simulink model "EcuAppM_StateMachine"  (R2022b)
settings: Solver=FixedStepDiscrete  StartTime=0  StopTime=50  FixedStep=1  RelTol=1e-3  EnableMultiTasking=on
values from neighbouring files (symbols this model uses):
  ECUAPPM_MAX_WAKEUP_SOURCES = mpt.Parameter    [EcuAppM_StateMachine_Param.m]    (also in EcuAppM_StateMachine_Param_For_Safety_Context.m)
  ECUAPPM_VALUE_ZERO = mpt.Parameter    [EcuAppM_StateMachine_Param.m]    (also in EcuAppM_StateMachine_Param_For_Safety_Context.m)
  EcuAppM_WakeupSourcesData = mpt.Parameter    [EcuAppM_StateMachine_Param.m]    (also in EcuAppM_StateMachine_Param_For_Safety_Context.m)
libraries: simulink x3
(part 2 of 2)

== stateflow chart EcuAppM_StateMachine/Subsystem/EcuAppM_StateChart ==
  state EcuAppM_WakeupValidationState
    entry:
    EcuAppM_WakeupValidationTimer = ECUAPPM_VALUE_ZERO;
    EcuAppMInfo.State  = eEcuAppM_WakeupValidation;
    EcuAppMInfo.CurrentJobStatus = ECUAPPM_JOB_IN_PROGRESS;
    EcuAppM_OnWakeupValidationWrapper(EcuAppM_BufferedWakeupSource);
    during:
    EcuAppMInfo.CurrentJobStatus = EcuAppM_ProcessJobStatusWrapper(EcuAppMInfo.State);
    EcuAppM_WakeupValidationTimer = EcuAppM_WakeupValidationTimer + ECUAPPM_PERIOD_MSEC;
    exit:
    EcuAppM_WakeupValidationTimer = ECUAPPM_VALUE_ZERO;
    EcuAppMInfo.CurrentJobStatus = ECUAPPM_JOB_IDLE;
  state EcuAppM_StartOfSleepTransientWrapper [function]
  state EcuAppM_PreGroupActivationState
    entry:
    EcuAppMInfo.State  = eEcuAppM_PreGroupActivation;
    EcuAppMInfo.CurrentJobStatus = ECUAPPM_JOB_IN_PROGRESS;
    EcuAppM_BufferedWakeupSource = EcuAppM_WakeupSource;
    EcuAppM_BufferedWakeupData = EcuAppM_ReadWakeupSourcesConfigData...
    (EcuAppM_BufferedWakeupSource);
    EcuAppM_OnStartupWrapper(EcuAppM_BufferedWakeupSource);
    during:
    EcuAppM_ProcessPreGroupsActivation(PRE_GROUP0);
    EcuAppMInfo.CurrentJobStatus = EcuAppM_ProcessJobStatusWrapper(EcuAppMInfo.State);
    exit:
    EcuAppMInfo.CurrentJobStatus = ECUAPPM_JOB_IDLE;
  state EcuAppM_StartPowerUpSequenceState
    entry:
    EcuAppMInfo.State  = eEcuAppM_StartPowerUpSequence;
    EcuAppMInfo.CurrentJobStatus = ECUAPPM_JOB_IN_PROGRESS;
    EcuAppM_OnPowerSeqStartWrapper(EcuAppMInfo.State);
    during:
    EcuAppMInfo.CurrentJobStatus = EcuAppM_ProcessJobStatusWrapper(EcuAppMInfo.State);
    exit:
    EcuAppMInfo.CurrentJobStatus = ECUAPPM_JOB_IDLE;
  state EcuAppM_ClearWakeupReasonWrapper [function]
  state EcuAppM_StartOfGroupsDeactivationWrapper [function]
  state EcuAppM_OnStartupWrapper(EcuAppM_BufferedWakeupSource) [function]
  state EcuAppM_ReadDataState
    entry:
    EcuAppMInfo.State  = eEcuAppM_ReadDataState;
    exit:
    EcuAppM_BufferedWakeupSource = EcuAppM_WakeupSource;
    state NVMReadallState [parallel]
      entry:
      EcuAppMInfo.CurrentJobStatus = ECUAPPM_JOB_IN_PROGRESS;
      EcuAppM_OnNVMReadAllWrapper(EcuAppM_BufferedWakeupSource);
      during:
      EcuAppMInfo.CurrentJobStatus = EcuAppM_ProcessJobStatusWrapper(EcuAppMInfo.State);
      exit:
      EcuAppMInfo.CurrentJobStatus = ECUAPPM_JOB_IDLE;
      settings: executionOrder=1
    state EcuAppM_PreGroup [parallel]
      entry:
      EcuAppM_ProcessPreGroupsActivation(PRE_GROUP1);
      during:
      EcuAppM_ProcessPreGroupsActivation(PRE_GROUP1);
      settings: executionOrder=2
  state EcuAppM_OnNVMReadAllWrapper(EcuAppM_BufferedWakeupSource) [function]
  state EcuAppM_OnWakeupValidationWrapper(EcuAppM_BufferedWakeupSource) [function]
  state EcuAppM_BackupDataWrapper [function]
  state EcuAppM_GroupsMgmtState
    note: Groups Activation and Deactivation stages summary:
        | 1.Once Deactivation started wake up request is accepted immedietly after ongoing group deactivation.
        | 2.Sleep request is accepted immedietly after ongoing group activation.
        | 3.While Partial wakeup groups are deactivating, if early wakeup comes should not consider immedietly.instead need to allow full deactivation of normal groups. Consider the early wakeup only from EcuAppM_BackupDataState .
        | This is to avoid unnecessary activation of not subcribed groups for that particular wakeup.
    state EcuAppM_GroupsActivationState
      entry:
      EcuAppMInfo.State  = eEcuAppM_GroupsActivation;
      EcuAppMInfo.CurrentJobStatus = ECUAPPM_JOB_IN_PROGRESS;
      during:
      EcuAppM_ProcessGroupsActivation(ECUAPPM_GROUP2,ECUAPPM_MAX_GROUPS - ECUAPPM_VALUE_ONE);
      EcuAppMInfo.CurrentJobStatus = EcuAppM_ProcessJobStatusWrapper(EcuAppMInfo.State);
      exit:
      EcuAppMInfo.CurrentJobStatus = ECUAPPM_JOB_IDLE;
    state EcuAppM_GroupsDeactivationState
      entry:
      EcuAppMInfo.State  = eEcuAppM_GroupsDeactivation;
      EcuAppMInfo.EarlyWakeupCheck = ECUAPPM_FALSE;
      EcuAppMInfo.CurrentJobStatus = ECUAPPM_JOB_IN_PROGRESS;
      EcuAppM_ClearWakeupReasonWrapper();
      EcuAppM_StartOfGroupsDeactivationWrapper();
      during:
      EcuAppM_ProcessGroupsDeactivation(ECUAPPM_MAX_GROUPS - ECUAPPM_VALUE_ONE,ECUAPPM_GROUP2,1);
      EcuAppMInfo.CurrentJobStatus = EcuAppM_ProcessJobStatusWrapper(EcuAppMInfo.State);
      exit:
      EcuAppMInfo.EarlyWakeupCheck = ECUAPPM_FALSE;
      EcuAppMInfo.CurrentJobStatus = ECUAPPM_JOB_IDLE;
    state EcuAppM_EarlyWakeupValidationState
      entry:
      EcuAppM_WakeupValidationTimer = ECUAPPM_VALUE_ZERO;
      EcuAppMInfo.State  = eEcuAppM_WakeupValidation;
      EcuAppMInfo.CurrentJobStatus = ECUAPPM_JOB_IN_PROGRESS;
      EcuAppM_BufferedWakeupData = EcuAppM_ReadWakeupSourcesConfigData(EcuAppM_BufferedWakeupSource);
      EcuAppM_OnWakeupValidationWrapper(EcuAppM_BufferedWakeupSource);
      EcuAppM_ClearWakeupReasonWrapper();
      during:
      EcuAppMInfo.CurrentJobStatus = EcuAppM_ProcessJobStatusWrapper(EcuAppMInfo.State);
      EcuAppM_WakeupValidationTimer = EcuAppM_WakeupValidationTimer + ECUAPPM_PERIOD_MSEC;
      exit:
      EcuAppM_WakeupValidationTimer = ECUAPPM_VALUE_ZERO;
      EcuAppMInfo.CurrentJobStatus = ECUAPPM_JOB_IDLE;
      EcuAppMInfo.EarlyWakeupCheck = ECUAPPM_FALSE;
    (default) -> EcuAppM_GroupsActivationState
    EcuAppM_GroupsActivationState -> EcuAppM_GroupsDeactivationState : [(EcuAppMInfo.CurrentJobStatus == ECUAPPM_JOB_DONE)&&(EcuAppM_CheckActivationStatetimerExpiry() == TRUE)&&...
        |  (EcuAppM_IsGroupsActivationDeactivationAllowed() == ECUAPPM_TRUE)&&(ApplicationSleepState == ECUAPPM_READY_TO_SLEEP)]
    EcuAppM_GroupsDeactivationState -> EcuAppM_EarlyWakeupValidationState [order 1] : [EcuAppMInfo.EarlyWakeupCheck  == ECUAPPM_TRUE]
    EcuAppM_EarlyWakeupValidationState -> EcuAppM_GroupsDeactivationState [order 1] : [(EcuAppMInfo.CurrentJobStatus == ECUAPPM_JOB_FAILED)||...
        |  (EcuAppM_WakeupValidationTimer >= EcuAppM_BufferedWakeupData.validationTime)]
    EcuAppM_EarlyWakeupValidationState -> EcuAppM_GroupsActivationState [order 2] : [(EcuAppMInfo.CurrentJobStatus == ECUAPPM_JOB_DONE)||...
        |  (EcuAppM_BufferedWakeupData.validationTime == ECUAPPM_VALIDATION_TIME_ZERO)]
  state EcuAppM_OnPowerSeqStartWrapper(State) [function]
  state EcuAppM_BufferedDataOutput = EcuAppM_ReadWakeupSourcesConfigData... [function]
    (EcuAppM_BufferedWakeupSource)
  state status = EcuAppM_ProcessJobStatusWrapper(state) [function]
    state status = EcuAppM_ProcessJobStatusFunc(state) [function]
    note: EcuAppM_ProcessJobStatusWrapper Summary:
        |
        | 1. EcuAppM_ProcessJobStatusWrapper Graphical function is used to trigger the EcuAppM_ProcessJobStatusFunc simulink Function.
        | 2.If we are calling EcuAppM_ProcessJobStatusFunc simulink Function With arguments directly, we are facing the error while generating the code(it seems to be a matlab issue).
        | 3.To avoid this, indirectly we are calling the sumulink function with arguments by using Graphical EcuAppM_ProcessJobStatusWrapper function.
        | 4.Calling Simulink function with arguments inside the graphical function is not giving any error hence currently following this approach.
    (default) -> (junction 2651)
    (junction 2651) -> (junction 2652) : {status = EcuAppM_ProcessJobStatusFunc(state)}
  state EcuAppM_BackupDataState
    entry:
    EcuAppMInfo.State  = eEcuAppM_BackupData;
    EcuAppMInfo.CurrentJobStatus = ECUAPPM_JOB_IN_PROGRESS;
    EcuAppM_BackupDataWrapper();
    during:
    EcuAppMInfo.CurrentJobStatus = EcuAppM_ProcessJobStatusWrapper(EcuAppMInfo.State);
    exit:
    EcuAppMInfo.CurrentJobStatus = ECUAPPM_JOB_IDLE;
  state EcuAppM_ProcessPreGroupsActivation(activationstage) [function]
    note: EcuAppM_ProcessPreGroupsActivation Summary:
        |
        | 1. This function will call EcuAppM_GroupsLifeCycleMgr for pre groups activation.Only for wakeup subscribed groups alone.
    (default) -> (junction 3283) : {
        |  pregrp0Index = ECUAPPM_VALUE_ZERO;
        |  pregrp1Index = ECUAPPM_VALUE_ZERO;
        | }
    (junction 3283) -> (junction 3401) [order 1] : [(activationstage == PRE_GROUP0)&&...
        |  (pregrp0Index < ECUAPPM_PREGROUP0_MAX_ELEMENTS)]
    (junction 3401) -> (junction 3284) [order 1] : [EcuAppM_PreGroup0Elements[pregrp0Index] < ECUAPPM_MAX_GROUPS]
    (junction 3284) -> (junction 3285) [order 1] : [((EcuAppM_GroupConfigData[EcuAppM_PreGroup0Elements[pregrp0Index]].wakeupSourceMask & EcuAppM_BufferedWakeupSource) == EcuAppM_BufferedWakeupSource)]
    (junction 3405) -> (junction 3283) : {
        |  pregrp0Index = pregrp0Index + ECUAPPM_VALUE_ONE;
        | }
    (junction 3283) -> (junction 3350) [order 2]
    (junction 3401) -> (junction 3405) [order 2]
    (junction 3284) -> (junction 3286) [order 2]
    (junction 3285) -> (junction 3287) : {
        |   EcuAppM_GroupsLifeCycleMgr(EcuAppM_PreGroup0Elements[pregrp0Index]);
        | }
    (junction 3286) -> (junction 3405)
    (junction 3287) -> (junction 3286)
    (junction 3350) -> (junction 3412) [order 1] : [(activationstage == PRE_GROUP1)&&...
        |  (pregrp1Index < ECUAPPM_PREGROUP1_MAX_ELEMENTS)]
    (junction 3412) -> (junction 3351) [order 1] : [EcuAppM_PreGroup1Elements[pregrp1Index] < ECUAPPM_MAX_GROUPS]
    (junction 3351) -> (junction 3352) [order 1] : [((EcuAppM_GroupConfigData[EcuAppM_PreGroup1Elements[pregrp1Index]].wakeupSourceMask & EcuAppM_BufferedWakeupSource) == EcuAppM_BufferedWakeupSource)]
    (junction 3414) -> (junction 3350) : {
        |  pregrp1Index = pregrp1Index + ECUAPPM_VALUE_ONE;
        | }
    (junction 3350) -> (junction 3362) [order 2]
    (junction 3412) -> (junction 3414) [order 2]
    (junction 3351) -> (junction 3361) [order 2]
    (junction 3352) -> (junction 3360) : {
        |   EcuAppM_GroupsLifeCycleMgr(EcuAppM_PreGroup1Elements[pregrp1Index]);
        | }
    (junction 3361) -> (junction 3414)
    (junction 3360) -> (junction 3361)
  state activationstatus = EcuAppM_IsPreGroupsActivated(activationstage) [function]
    note: EcuAppM_IsPreGroupsActivated Summary:
        |
        | 1. This function is to confirm pre-stages groups are completly activated or not(only particular wakeup subscribed groups status should be checked).
    (default) -> (junction 3223) : {
        |  pregrp0Index = ECUAPPM_VALUE_ZERO;
        |  pregrp1Index = ECUAPPM_VALUE_ZERO;
        | }
    (junction 3336) -> (junction 3419) [order 1] : [EcuAppM_PreGroup0Elements[pregrp0Index] < ECUAPPM_MAX_GROUPS]
    (junction 3419) -> (junction 3224) [order 1] : [((EcuAppM_GroupConfigData[EcuAppM_PreGroup0Elements[pregrp0Index]].wakeupSourceMask & EcuAppM_BufferedWakeupSource) == EcuAppM_BufferedWakeupSource)]
    (junction 3224) -> (junction 3225) [order 1] : [EcuAppM_GroupsInfo.GroupState[EcuAppM_PreGroup0Elements[pregrp0Index]] == eGroup_StateActive]
    (junction 3223) -> (junction 3336) [order 1] : [(activationstage == PRE_GROUP0)&&...
        |  (pregrp0Index < ECUAPPM_PREGROUP0_MAX_ELEMENTS)]
    (junction 3338) -> (junction 3223)
    (junction 3223) -> (junction 3368) [order 2]
    (junction 3336) -> (junction 3338) [order 2] : {
        |  pregrp0Index = pregrp0Index + ECUAPPM_VALUE_ONE;
        |  activationstatus = ECUAPPM_TRUE;
        | }
    (junction 3419) -> (junction 3421) [order 2] : {
        |  pregrp0Index = pregrp0Index + ECUAPPM_VALUE_ONE;
        |  activationstatus = ECUAPPM_TRUE;
        | }
    (junction 3225) -> (junction 3228) : {
        |  pregrp0Index = pregrp0Index + ECUAPPM_VALUE_ONE;
        |  activationstatus = ECUAPPM_TRUE;
        | }
    (junction 3224) -> (junction 3227) [order 2] : {
        |   pregrp0Index = ECUAPPM_PREGROUP0_MAX_ELEMENTS;
        |   activationstatus = ECUAPPM_FALSE;
        | }
    (junction 3421) -> (junction 3338)
    (junction 3227) -> (junction 3421)
    (junction 3228) -> (junction 3227)
    (junction 3368) -> (junction 3424) [order 1] : [(activationstage == PRE_GROUP1)&&...
        |  (pregrp1Index < ECUAPPM_PREGROUP1_MAX_ELEMENTS)]
    (junction 3424) -> (junction 3382) [order 1] : [EcuAppM_PreGroup1Elements[pregrp0Index] < ECUAPPM_MAX_GROUPS]
    (junction 3382) -> (junction 3369) [order 1] : [((EcuAppM_GroupConfigData[EcuAppM_PreGroup1Elements[pregrp0Index]].wakeupSourceMask & EcuAppM_BufferedWakeupSource) == EcuAppM_BufferedWakeupSource)]
    (junction 3369) -> (junction 3367) [order 1] : [EcuAppM_GroupsInfo.GroupState[EcuAppM_PreGroup1Elements[pregrp0Index]] == eGroup_StateActive]
    (junction 3426) -> (junction 3368)
    (junction 3369) -> (junction 3371) [order 2] : {
        |   pregrp1Index = ECUAPPM_PREGROUP1_MAX_ELEMENTS;
        |   activationstatus = ECUAPPM_FALSE;
        | }
    (junction 3368) -> (junction 3370) [order 2]
    (junction 3424) -> (junction 3426) [order 2] : {
        |  pregrp1Index = pregrp1Index + ECUAPPM_VALUE_ONE;
        |  activationstatus = ECUAPPM_TRUE;
        | }
    (junction 3382) -> (junction 3381) [order 2] : {
        |  pregrp1Index = pregrp1Index + ECUAPPM_VALUE_ONE;
        |  activationstatus = ECUAPPM_TRUE;
        | }
    (junction 3367) -> (junction 3372) : {
        |   pregrp1Index = pregrp1Index + ECUAPPM_VALUE_ONE;
        |   activationstatus = ECUAPPM_TRUE;
        | }
    (junction 3381) -> (junction 3426)
    (junction 3371) -> (junction 3381)
    (junction 3372) -> (junction 3371)
  state EcuAppM_StartPowerDownSequenceState
    entry:
    EcuAppMInfo.State  = eEcuAppM_StartPowerDownSequence;
    EcuAppMInfo.CurrentJobStatus = ECUAPPM_JOB_IN_PROGRESS;
    EcuAppM_OnPowerSeqStartWrapper(EcuAppMInfo.State);
    during:
    EcuAppMInfo.CurrentJobStatus = EcuAppM_ProcessJobStatusWrapper(EcuAppMInfo.State);
    exit:
    EcuAppMInfo.CurrentJobStatus = ECUAPPM_JOB_IDLE;
  state EcuAppM_ProcessGroupsActivation( From_groupid,To_groupid) [function]
    note: EcuAppM_ProcessGroupsActivation Summary:
        |
        | 1. This function is used to call the EcuAppM_GroupsLifeCycleMgr for particular wakup subscribed groups alone.
        | 2. Groups can be activated ASYNCHRONUS or SYNCHRONUS based on the ECUAPPM_GROUP_ACTIVATION_TYPE
        | configuration.
    (default) -> (junction 2493) : {
        |  groupId = From_groupid;
        |  group_limit = To_groupid;
        | }
    (junction 2493) -> (junction 2494) [order 1] : [(groupId <= group_limit)&&...
        | (ECUAPPM_GROUP_ACTIVATION_TYPE == ASYNCHRONUS)]
    (junction 2494) -> (junction 2495) [order 1] : [((EcuAppM_GroupConfigData[groupId].wakeupSourceMask & EcuAppM_BufferedWakeupSource) == EcuAppM_BufferedWakeupSource)]
    (junction 2500) -> (junction 2493)
    (junction 2493) -> (junction 2499) [order 2]
    (junction 2494) -> (junction 2500) [order 2] : {groupId = groupId + ECUAPPM_VALUE_ONE;}
    (junction 2495) -> (junction 2534) : {
        |   EcuAppM_GroupsLifeCycleMgr(groupId);
        |   groupId = groupId + ECUAPPM_VALUE_ONE;
        | }
    (junction 2534) -> (junction 2500)
    (junction 2499) -> (junction 2536) [order 1] : [(groupId <= group_limit)&&...
        | (ECUAPPM_GROUP_ACTIVATION_TYPE == SYNCHRONUS)]
    (junction 2536) -> (junction 2550) [order 1] : [((EcuAppM_GroupConfigData[groupId].wakeupSourceMask & EcuAppM_BufferedWakeupSource) == EcuAppM_BufferedWakeupSource)&&...
        | (EcuAppM_GroupsInfo.GroupState[groupId] != eGroup_StateActive)]
    (junction 2539) -> (junction 2499) : {groupId = groupId + ECUAPPM_VALUE_ONE;}
    (junction 2499) -> (junction 2541) [order 2]
    (junction 2536) -> (junction 2539) [order 2]
    (junction 2550) -> (junction 2662) : {
        |   EcuAppM_GroupsLifeCycleMgr(groupId);
        | }
    (junction 2662) -> (junction 2661) [order 1] : [EcuAppM_GroupsInfo.GroupState[groupId] == eGroup_StateActive]
    (junction 2661) -> (junction 2668)
    (junction 2662) -> (junction 2665) [order 2]
    (junction 2668) -> (junction 2539)
    (junction 2665) -> (junction 2541)
  state EcuAppM_GroupsLifeCycleMgr(groupId) [function]
    state EcuAppM_FailSafeMechanismWrapper(index,status) [function]
    state EcuAppM_ReturnValue = EcuAppM_GroupStateChangeRequestWrapper(groupId,StateCmd) [function]
    state EcuAppM_ReturnValue = EcuAppM_SafeGroupStateChangeRequestWrapper(groupId,StateCmd) [function]
    state EcuAppM_GroupStatusChangeCbkWrapper(index,status) [function]
    state EcuAppM_GroupActivationAllowed = EcuAppM_GroupActivationCalloutWrapper(unit8_t) [function]
    note: EcuAppM_GroupsLifeCycleMgr summary:
        |
        | 1.This function is used to send the group state change request for different states (eGroup_StateInit,eGroup_StateActivation,eGroup_StateActive and eGroup_StateDeactivation) .
        | 2. If the state is not changed with in configured time then fail safe action call is triggered.
    (default) -> (junction 3156)
    (junction 3155) -> (junction 3160) [order 1] : [(EcuAppMInfo.State != eEcuAppM_GroupsDeactivation)&&(EcuAppMInfo.State != eEcuAppM_PreGroupDeactivation)]
    (junction 3156) -> (junction 3155) [order 1] : [EcuAppM_GroupsInfo.GroupState[groupId] == eGroup_StateOff]
    (junction 3160) -> (junction 3162) : {
        |   EcuAppM_GroupsInfo.GroupState[groupId] = eGroup_StateInit;
        | }
    (junction 3156) -> (junction 2676) [order 2]
    (junction 3155) -> (junction 3164) [order 2]
    (junction 3164) -> (junction 3162)
    (junction 3162) -> (junction 3170)
    (junction 3170) -> (junction 2685)
    (junction 2676) -> (junction 3436) [order 1] : [EcuAppM_GroupsInfo.GroupState[groupId] == eGroup_StateInit]
    (junction 3436) -> (junction 2677) [order 1] : [(EcuAppM_GroupConfigData[groupId].safetyLevel > eSafetyLevel_QM)]
    (junction 2676) -> (junction 2691) [order 2]
    (junction 3436) -> (junction 3435) [order 2] : {
        |  ReturnStatus = EcuAppM_GroupStateChangeRequestWrapper(groupId,eGroup_StateInit);
        | }
    (junction 2677) -> (junction 2680) : {
        |  ReturnStatus = EcuAppM_SafeGroupStateChangeRequestWrapper(groupId,eGroup_StateInit);
        | }
    (junction 3435) -> (junction 2680)
    (junction 2681) -> (junction 3507) [order 1] : [EcuAppM_GroupActivationCalloutWrapper(groupId) == ECUAPPM_TRUE]
    (junction 2680) -> (junction 2681) [order 1] : [ReturnStatus == ECUAPPM_JOB_DONE]...
        | {EcuAppM_GroupStatusChangeCbkWrapper(groupId,EcuAppM_GroupsInfo.GroupState[groupId]);
        |   EcuAppM_GroupsInfo.GroupActivityTimer[groupId]  = ECUAPPM_VALUE_ZERO;}
    (junction 2681) -> (junction 2927) [order 2] : {
        |   EcuAppM_GroupsInfo.GroupState[groupId] = eGroup_StateInactive;
        | }
    (junction 3507) -> (junction 3508) : {
        |   EcuAppM_GroupsInfo.GroupState[groupId] = eGroup_StateActivation;
        | }
    (junction 2680) -> (junction 2682) [order 2] : {
        |  EcuAppM_GroupsInfo.GroupActivityTimer[groupId] += ECUAPPM_PERIOD_MSEC;
        | }
    (junction 2927) -> (junction 3508)
    (junction 3508) -> (junction 2685)
    (junction 2685) -> (junction 2690)
    (junction 2682) -> (junction 2683) [order 1] : [ EcuAppM_GroupsInfo.GroupActivityTimer[groupId] >= EcuAppM_GroupConfigData[groupId].failSafeTimeout ]
    (junction 2682) -> (junction 2688) [order 2]
    (junction 2683) -> (junction 2925) : {
        |  EcuAppM_FailSafeMechanismWrapper(groupId,EcuAppM_GroupsInfo.GroupState[groupId]);
        | }
    (junction 2688) -> (junction 2925)
    (junction 2925) -> (junction 2690)
    (junction 2690) -> (junction 2698)
    (junction 2691) -> (junction 3449) [order 1] : [EcuAppM_GroupsInfo.GroupState[groupId] == eGroup_StateActivation]
    (junction 3449) -> (junction 2692) [order 1] : [(EcuAppM_GroupConfigData[groupId].safetyLevel > eSafetyLevel_QM)]
    (junction 2691) -> (junction 3174) [order 2]
    (junction 3449) -> (junction 3451) [order 2] : {
        |  ReturnStatus = EcuAppM_GroupStateChangeRequestWrapper(groupId,eGroup_StateActivation);
        | }
    (junction 2692) -> (junction 2693) : {
        |  ReturnStatus = EcuAppM_SafeGroupStateChangeRequestWrapper(groupId,eGroup_StateActivation);
        | }
    (junction 3451) -> (junction 2693)
    (junction 2693) -> (junction 2694) [order 1] : [ReturnStatus == ECUAPPM_JOB_DONE]
    (junction 2693) -> (junction 2695) [order 2] : {
        |  EcuAppM_GroupsInfo.GroupActivityTimer[groupId] += ECUAPPM_PERIOD_MSEC;
        | }
    (junction 2694) -> (junction 2697) : {
        |  EcuAppM_GroupStatusChangeCbkWrapper(groupId,EcuAppM_GroupsInfo.GroupState[groupId]);
        |  EcuAppM_GroupsInfo.GroupActivityTimer[groupId]  = ECUAPPM_VALUE_ZERO;
        |  EcuAppM_GroupsInfo.GroupState[groupId] = eGroup_StateActive;
        | }
    (junction 2695) -> (junction 2696) [order 1] : [ EcuAppM_GroupsInfo.GroupActivityTimer[groupId] >= EcuAppM_GroupConfigData[groupId].failSafeTimeout ]
    (junction 2697) -> (junction 2698)
    (junction 2695) -> (junction 2699) [order 2]
    (junction 2696) -> (junction 2700) : {
        |  EcuAppM_FailSafeMechanismWrapper(groupId,EcuAppM_GroupsInfo.GroupState[groupId]);
        | }
    (junction 2698) -> (junction 2701)
    (junction 2699) -> (junction 2700)
    (junction 2700) -> (junction 2701)
    (junction 2701) -> (junction 3185)
    (junction 3174) -> (junction 3466) [order 1] : [EcuAppM_GroupsInfo.GroupState[groupId] == eGroup_StateActive]
    (junction 3466) -> (junction 3178) [order 1] : [(EcuAppMInfo.State == eEcuAppM_GroupsDeactivation)||(EcuAppMInfo.State == eEcuAppM_PreGroupDeactivation)]
    (junction 3174) -> (junction 2702) [order 2]
    (junction 3466) -> (junction 3468) [order 2]
    (junction 3178) -> (junction 3470)
    (junction 3468) -> (junction 3470) [order 1] : [(EcuAppM_GroupActivationCalloutWrapper(groupId) != ECUAPPM_TRUE)]
    (junction 3468) -> (junction 3182) [order 2]
    (junction 3470) -> (junction 3180) : {
        |  EcuAppM_GroupsInfo.GroupState[groupId] = eGroup_StateDeactivation;
        | }
    (junction 3182) -> (junction 3180)
    (junction 3180) -> (junction 3185)
    (junction 3185) -> (junction 2710)
    (junction 2702) -> (junction 3454) [order 1] : [EcuAppM_GroupsInfo.GroupState[groupId] == eGroup_StateDeactivation]
    (junction 3454) -> (junction 2704) [order 1] : [(EcuAppM_GroupConfigData[groupId].safetyLevel > eSafetyLevel_QM)]
    (junction 2702) -> (junction 3484) [order 2]
    (junction 3454) -> (junction 3456) [order 2] : {
        |   ReturnStatus = EcuAppM_GroupStateChangeRequestWrapper(groupId,eGroup_StateDeactivation);
        | }
    (junction 2704) -> (junction 2705) : {
        |   ReturnStatus = EcuAppM_SafeGroupStateChangeRequestWrapper(groupId,eGroup_StateDeactivation);
        | }
    (junction 3456) -> (junction 2705)
    (junction 2705) -> (junction 2706) [order 1] : [ReturnStatus == ECUAPPM_JOB_DONE]
    (junction 2705) -> (junction 2707) [order 2] : {
        |  EcuAppM_GroupsInfo.GroupActivityTimer[groupId] += ECUAPPM_PERIOD_MSEC;
        | }
    (junction 2706) -> (junction 2709) : {
        |  EcuAppM_GroupStatusChangeCbkWrapper(groupId,EcuAppM_GroupsInfo.GroupState[groupId]);
        |  EcuAppM_GroupsInfo.GroupActivityTimer[groupId]  = ECUAPPM_VALUE_ZERO;
        |  EcuAppM_GroupsInfo.GroupState[groupId] = eGroup_StateInactive;
        | }
    (junction 2707) -> (junction 2708) [order 1] : [ EcuAppM_GroupsInfo.GroupActivityTimer[groupId] >= EcuAppM_GroupConfigData[groupId].failSafeTimeout ]
    (junction 2709) -> (junction 2710)
    (junction 2707) -> (junction 2712) [order 2]
    (junction 2710) -> (junction 2714)
    (junction 2708) -> (junction 2713) : {
        |  EcuAppM_GroupsInfo.GroupState[groupId] = eGroup_StateInactive;
        |  EcuAppM_GroupsInfo.GroupActivityTimer[groupId]  = ECUAPPM_VALUE_ZERO;
        |  EcuAppM_FailSafeMechanismWrapper(groupId,EcuAppM_GroupsInfo.GroupState[groupId]);
        | }
    (junction 2712) -> (junction 2713)
    (junction 2713) -> (junction 2714)
    (junction 2714) -> (junction 3497)
    (junction 3484) -> (junction 3487) [order 1] : [EcuAppM_GroupsInfo.GroupState[groupId] == eGroup_StateInactive]
    (junction 3487) -> (junction 3489) [order 1] : [(EcuAppMInfo.State != eEcuAppM_GroupsDeactivation)&&...
        |  (EcuAppMInfo.State != eEcuAppM_PreGroupDeactivation)&&...
        |  (EcuAppM_GroupActivationCalloutWrapper(groupId) == ECUAPPM_TRUE)]
    (junction 3484) -> (junction 2715) [order 2]
    (junction 3487) -> (junction 3492) [order 2]
    (junction 3489) -> (junction 3494) : {
        |   EcuAppM_GroupsInfo.GroupState[groupId] = eGroup_StateActivation;
        | }
    (junction 3492) -> (junction 3494)
    (junction 3494) -> (junction 3497)
    (junction 3497) -> (junction 2716)
    (junction 2716) -> (junction 2715)
    (junction 2715) -> (junction 2717)
  state activationdeactivationAllowed = EcuAppM_IsGroupsActivationDeactivationAllowed [function]
    note: EcuAppM_IsGroupsActivationDeactivationAllowed Summary:
        |
        | 1.This function is used to know whther groups are allowed to deactivate or not. Groups either should be in active state or should be in inactive state.
        | Then only based on Application sleep status will allow for groups deactivation.
    (default) -> (junction 3047) : {
        | groupId =ECUAPPM_VALUE_ZERO;
        | activationdeactivationAllowed = ECUAPPM_FALSE;
        | }
    (junction 3047) -> (junction 3048) [order 1] : [groupId < ECUAPPM_MAX_GROUPS]
    (junction 3048) -> (junction 3049) [order 1] : [(EcuAppM_GroupsInfo.GroupState[groupId] == eGroup_StateActive)||...
        |  (EcuAppM_GroupsInfo.GroupState[groupId] == eGroup_StateInactive)||...
        |  (EcuAppM_GroupsInfo.GroupState[groupId] == eGroup_StateOff)]
    (junction 3050) -> (junction 3047)
    (junction 3047) -> (junction 3052) [order 2]
    (junction 3048) -> (junction 3050) [order 2] : {
        | groupId = ECUAPPM_MAX_GROUPS;
        | activationdeactivationAllowed = ECUAPPM_FALSE;
        | }
    (junction 3049) -> (junction 3051) : {
        |  groupId = groupId + ECUAPPM_VALUE_ONE;
        |  activationdeactivationAllowed = ECUAPPM_TRUE;
        | }
    (junction 3051) -> (junction 3050)
  state EcuAppM_PreGroupDeactivationState
    entry:
    EcuAppMInfo.State  = eEcuAppM_PreGroupDeactivation;
    EcuAppMInfo.CurrentJobStatus = ECUAPPM_JOB_IN_PROGRESS;
    during:
    EcuAppM_ProcessGroupsDeactivation(ECUAPPM_GROUP1,ECUAPPM_GROUP0,0);
    EcuAppMInfo.CurrentJobStatus =EcuAppM_ProcessJobStatusWrapper(EcuAppMInfo.State);
    exit:
    EcuAppMInfo.CurrentJobStatus = ECUAPPM_JOB_IDLE;
  state EcuAppM_SleepTransientState
    entry:
    EcuAppMInfo.State  = eEcuAppM_SleepTransient;
    EcuAppM_ClearWakeupReasonWrapper();
    EcuAppM_StartOfSleepTransientWrapper();
    during:
    EcuAppMInfo.CurrentJobStatus = EcuAppM_ProcessJobStatusWrapper(EcuAppMInfo.State);
    exit:
    EcuAppMInfo.CurrentJobStatus = ECUAPPM_JOB_IDLE;
  state deactivationStatus = EcuAppM_GroupsDeactivationStatus(From_groupid,To_groupid) [function]
    note: EcuAppM_GroupsDeactivationStatus Summary:
        |
        | 1.This function is used to know groups are completly deactivated or not.
    (default) -> (junction 3018) : {
        | groupId = From_groupid;
        | group_limit = To_groupid;
        | deactivationStatus = ECUAPPM_FALSE;
        | }
    (junction 3018) -> (junction 3019) [order 1] : [groupId <=group_limit]
    (junction 3019) -> (junction 3020) [order 1] : [(EcuAppM_GroupsInfo.GroupState[groupId] == eGroup_StateInactive)||...
        |  (EcuAppM_GroupConfigData[groupId].deactivationType == KEEP_ALIVE)||...
        | (EcuAppM_GroupsInfo.GroupState[groupId] == eGroup_StateOff)]
    (junction 3021) -> (junction 3018)
    (junction 3018) -> (junction 3023) [order 2]
    (junction 3019) -> (junction 3021) [order 2] : {
        |  groupId = group_limit+1;
        |  deactivationStatus = ECUAPPM_FALSE;
        | }
    (junction 3020) -> (junction 3022) : {
        |  groupId = groupId + ECUAPPM_VALUE_ONE;
        |  deactivationStatus = ECUAPPM_TRUE;
        | }
    (junction 3022) -> (junction 3021)
  state EcuAppM_ProcessGroupsDeactivation(From_groupid,To_groupid,... [function]
    EarlyWakeupNecessity)
    note: EcuAppM_ProcessGroupsDeactivation Summary:
        |
        | 1.This function will call EcuAppM_GroupsLifeCycleMgr for deactvating the groups. This is triggered from deactivation stages of statemachine.
        | 2.Groups Deactivation performed from higer index group to lower index group inorder to avoid the dependancies b/w the groups.
        | 3.After Complete Deactivation of individual group allowing next group to Deactive otherwise keep on calling EcuAppM_ActivateDeactivategrps() Function until respective group deactivation completion.
        | 4. EcuAppM_WakeupSource is checked immedielty after complete deactivation of particular group. if wakeup event exist then moving to group activation state. Other wise proceeding to deactvate other activated groups.
        | 5. EarlyWakeupNecessity flag it used to identify to allow early wakeup or not. This flag is necessary to avoid early wakeup after EcuAppM_BackupDataState . If early wakeup comes after EcuAppM_BackupDataState we are allowing to go complete sleep then wakeup.
    (default) -> (junction 3067) : {
        | groupId = From_groupid;
        | group_limit = To_groupid;
        | }
    (junction 3067) -> (junction 3068) [order 1] : [groupId >= group_limit]
    (junction 3068) -> (junction 3069) [order 1] : [EcuAppM_GroupConfigData[groupId].deactivationType == SHUTDOWN]
    (junction 3069) -> (junction 3146) [order 1] : [(EcuAppM_WakeupSource != ECUAPPM_NOWKPEVENT)&&...
        |  (ECUAPPM_TRUE == EcuAppM_IsGroupsActivationDeactivationAllowed())&&...
        |  (EcuAppM_BufferedWakeupData.wakeupReaction!= PARTIAL)&&...
        |  (EarlyWakeupNecessity == ECUAPPM_TRUE )]
    (junction 3070) -> (junction 3067) : {groupId = groupId - ECUAPPM_VALUE_ONE;}
    (junction 3146) -> (junction 3148) : {
        |  EcuAppMInfo.EarlyWakeupCheck = ECUAPPM_TRUE;
        |  EcuAppM_BufferedWakeupSource = EcuAppM_WakeupSource;
        | }
    (junction 3068) -> (junction 3120) [order 2]
    (junction 3069) -> (junction 3634) [order 2] : {
        |  EcuAppM_GroupsLifeCycleMgr(groupId);
        | }
    (junction 3067) -> (junction 3073) [order 2]
    (junction 3120) -> (junction 3070) [order 1] : [groupId >= ECUAPPM_VALUE_ONE]
    (junction 3634) -> (junction 3120) [order 1] : [(EcuAppM_GroupsInfo.GroupState[groupId] == eGroup_StateInactive)||...
        |  (EcuAppM_GroupsInfo.GroupState[groupId] == eGroup_StateOff)]
    (junction 3120) -> (junction 3122) [order 2]
    (junction 3634) -> (junction 3074) [order 2]
    (junction 3122) -> (junction 3073)
    (junction 3074) -> (junction 3122)
    (junction 3148) -> (junction 3074)
  state EcuAppM_IsActivationTimerExpired = EcuAppM_CheckActivationStatetimerExpiry [function]
    (default) -> (junction 3587)
    (junction 3587) -> (junction 3589) [order 1] : [ECUAPPM_MIN_GROUP_ACTIVE_TIME != ECUAPPM_VALUE_ZERO ]
    (junction 3589) -> (junction 3595) [order 1] : [EcuAppMActivationTimer >= ECUAPPM_MIN_GROUP_ACTIVE_TIME]
    (junction 3587) -> (junction 3591) [order 2] : {
        |      EcuAppM_IsActivationTimerExpired = TRUE;
        | }
    (junction 3589) -> (junction 3593) [order 2] : {
        |  EcuAppMActivationTimer = EcuAppMActivationTimer+ECUAPPM_PERIOD_MSEC;
        |  EcuAppM_IsActivationTimerExpired = FALSE;
        | }
    (junction 3595) -> (junction 3597) : {
        | EcuAppM_IsActivationTimerExpired = TRUE;
        | EcuAppMActivationTimer = 0;
        | }
    (junction 3593) -> (junction 3597)
    (junction 3597) -> (junction 3614)
    (junction 3614) -> (junction 3591)
    (junction 3591) -> (junction 3613)
  state EcuAppM_InitState
    entry:
    EcuAppMInfo.State = eEcuAppM_Init;
    EcuAppMInfo.CurrentJobStatus = ECUAPPM_JOB_IDLE;
  state EcuAppM_SleepState
    entry:
    EcuAppMInfo.State  = eEcuAppM_SleepState;
    EcuAppMInfo.CurrentJobStatus = ECUAPPM_JOB_IN_PROGRESS;
    during:
    EcuAppMInfo.CurrentJobStatus = EcuAppM_ProcessJobStatusWrapper(EcuAppMInfo.State);
    exit:
    EcuAppMInfo.CurrentJobStatus = ECUAPPM_JOB_IDLE;
  EcuAppM_BackupDataState -> EcuAppM_EarlyWakeupValidationState [order 1] : [(EcuAppM_WakeupSource != ECUAPPM_NOWKPEVENT)&&...
      |  (EcuAppMInfo.CurrentJobStatus == ECUAPPM_JOB_DONE)]
      | {EcuAppM_BufferedWakeupSource = EcuAppM_WakeupSource;
      |   EcuAppMInfo.EarlyWakeupCheck = ECUAPPM_TRUE;}
  EcuAppM_GroupsDeactivationState -> EcuAppM_BackupDataState [order 2] : [((EcuAppMInfo.CurrentJobStatus == ECUAPPM_JOB_DONE))&&...
      |  (EcuAppM_GroupsDeactivationStatus(ECUAPPM_GROUP2,ECUAPPM_MAX_GROUPS - ECUAPPM_VALUE_ONE) == ECUAPPM_TRUE)]
  EcuAppM_PreGroupActivationState -> EcuAppM_WakeupValidationState [order 2] : [(EcuAppMInfo.CurrentJobStatus == ECUAPPM_JOB_DONE) &&...
      |  (EcuAppM_BufferedWakeupData.validationTime != ECUAPPM_VALIDATION_TIME_ZERO)&&...
      |  (EcuAppM_IsPreGroupsActivated(PRE_GROUP0) == ECUAPPM_TRUE)]
  EcuAppM_WakeupValidationState -> EcuAppM_StartPowerUpSequenceState [order 1] : [EcuAppMInfo.CurrentJobStatus == ECUAPPM_JOB_DONE]
  EcuAppM_WakeupValidationState -> EcuAppM_SleepTransientState [order 2] : [(EcuAppMInfo.CurrentJobStatus == ECUAPPM_JOB_FAILED)||...
      |  (EcuAppM_WakeupValidationTimer >= EcuAppM_BufferedWakeupData.validationTime)]
  EcuAppM_PreGroupActivationState -> EcuAppM_StartPowerUpSequenceState [order 1] : [(EcuAppMInfo.CurrentJobStatus == ECUAPPM_JOB_DONE) &&...
      |  (EcuAppM_BufferedWakeupData.validationTime == ECUAPPM_VALIDATION_TIME_ZERO)&&...
      |  (EcuAppM_IsPreGroupsActivated(PRE_GROUP0) == ECUAPPM_TRUE)]
  EcuAppM_StartPowerUpSequenceState -> EcuAppM_ReadDataState : [EcuAppMInfo.CurrentJobStatus == ECUAPPM_JOB_DONE]
  EcuAppM_InitState -> EcuAppM_PreGroupActivationState : [EcuAppM_WakeupSource != ECUAPPM_NOWKPEVENT]
  (junction 3563) -> EcuAppM_PreGroupActivationState [order 1] : [EcuAppM_WakeupSource != ECUAPPM_NOWKPEVENT]
  EcuAppM_SleepState -> EcuAppM_PreGroupActivationState [order 1] : [(EcuAppMInfo.CurrentJobStatus == ECUAPPM_JOB_DONE)&&...
      |  (EcuAppM_WakeupSource != ECUAPPM_NOWKPEVENT)]
  EcuAppM_ReadDataState -> EcuAppM_GroupsMgmtState : [(EcuAppMInfo.CurrentJobStatus == ECUAPPM_JOB_DONE)&&...
      |  (EcuAppM_IsPreGroupsActivated(PRE_GROUP1) == ECUAPPM_TRUE)]
  (default) -> (junction 3563) : {
      | EcuAppMInfo.State = eEcuAppM_Init;
      | EcuAppMInfo.CurrentJobStatus = ECUAPPM_JOB_IDLE;
      | }
  (junction 3563) -> EcuAppM_InitState [order 2]
  EcuAppM_BackupDataState -> EcuAppM_StartPowerDownSequenceState [order 2] : [EcuAppMInfo.CurrentJobStatus == ECUAPPM_JOB_DONE]
  EcuAppM_StartPowerDownSequenceState -> EcuAppM_PreGroupDeactivationState : [EcuAppMInfo.CurrentJobStatus == ECUAPPM_JOB_DONE]
  EcuAppM_SleepTransientState -> EcuAppM_PreGroupDeactivationState : [EcuAppMInfo.CurrentJobStatus == ECUAPPM_JOB_DONE]
  EcuAppM_PreGroupDeactivationState -> EcuAppM_SleepState : [(EcuAppMInfo.CurrentJobStatus == ECUAPPM_JOB_DONE)&&...
      |  (EcuAppM_GroupsDeactivationStatus(ECUAPPM_GROUP0,ECUAPPM_GROUP1) == ECUAPPM_TRUE)]
  EcuAppM_SleepState -> EcuAppM_InitState [order 2] : [EcuAppMInfo.CurrentJobStatus == ECUAPPM_JOB_DONE]
  data: EcuAppM_BufferedWakeupSource function_input uint32 size=1; EcuAppM_BufferedWakeupSource function_input uint32 size=1; EcuAppM_BufferedWakeupSource function_input uint32 size=1; State function_input uint8 size=1; EcuAppM_BufferedWakeupSource function_input uint32 size=1; EcuAppM_BufferedDataOutput function_output Bus: EcuAppM_WakeupSourcesType size=1; state function_input uint8 size=1; status function_output uint8 size=1; state function_input uint8; status function_output uint8; activationstage function_input uint8; pregrp0Index local uint8; pregrp1Index local uint8; activationstatus function_output uint8; activationstage function_input uint8; pregrp0Index local uint8; pregrp1Index local uint8; groupId local uint8; From_groupid function_input uint8; To_groupid function_input uint8; group_limit local uint8; index function_input uint8 size=1; status function_input uint8 size=1; groupId function_input uint8 size=1; EcuAppM_ReturnValue function_output; StateCmd function_input uint8 size=1; groupId function_input uint8 size=1; EcuAppM_ReturnValue function_output; StateCmd function_input uint8 size=1; index function_input uint8 size=1; status function_input uint8 size=1; unit8_t function_input uint8 size=1; EcuAppM_GroupActivationAllowed function_output; groupId function_input uint8; ReturnStatus local uint8; groupId local uint8; activationdeactivationAllowed function_output uint8; From_groupid function_input uint8; deactivationStatus function_output uint8; groupId local uint8; To_groupid function_input uint8; group_limit local uint8; groupId local uint8; From_groupid function_input uint8; To_groupid function_input uint8; group_limit local uint8; EarlyWakeupNecessity function_input uint8; EcuAppM_IsActivationTimerExpired function_output uint8; ECUAPPM_VALIDATION_SUCESS parameter uint8; ECUAPPM_VALIDATION_FAILED parameter uint8; ApplicationSleepState input uint8; ECUAPPM_PERIOD_MSEC parameter uint16; ECUAPPM_NOWKPEVENT parameter uint8; ECUAPPM_READY_TO_SLEEP parameter uint8; ECUAPPM_VALIDATION_TIME_ZERO parameter uint8; ECUAPPM_TRUE parameter uint8; ECUAPPM_REFUSE_TO_SLEEP parameter uint8; ECUAPPM_FALSE parameter uint8; ECUAPPM_VALUE_ONE parameter uint8; ECUAPPM_GROUP1 parameter uint8; ECUAPPM_GROUP0 parameter uint8; SYNCHRONUS parameter uint8; ECUAPPM_MAX_GROUPS parameter uint8; EcuAppM_GroupsInfo local Bus: EcuAppM_GroupsInfo; EcuAppMInfo output Bus: EcuAppMInfo; EcuAppM_WakeupValidationTimer local double [0..500]; ECUAPPM_VALUE_ZERO parameter uint8; ASYNCHRONUS parameter uint8; EcuAppM_GroupConfigData parameter Bus: EcuAppM_GroupConfigType; EcuAppM_WakeupSource input uint32; SHUTDOWN parameter uint8; ECUAPPM_JOB_IDLE parameter uint8; ECUAPPM_JOB_IN_PROGRESS parameter uint8; ECUAPPM_JOB_DONE parameter uint8; ECUAPPM_JOB_FAILED parameter uint8; KEEP_ALIVE parameter uint8; ECUAPPM_GROUP2 parameter uint8; ECUAPPM_MAX_WAKEUP_SOURCES parameter uint16; EcuAppM_WakeupSourcesData parameter Bus: EcuAppM_WakeupSourcesType; EcuAppM_BufferedWakeupSource local double; FULL parameter uint8; PARTIAL parameter uint8; EcuAppM_BufferedWakeupData local double; PRE_GROUP1 parameter uint8; PRE_GROUP0 parameter uint8; ECUAPPM_PREGROUP1_MAX_ELEMENTS parameter uint8; ECUAPPM_PREGROUP0_MAX_ELEMENTS parameter uint8; EcuAppM_PreGroup0Elements parameter uint8; EcuAppM_PreGroup1Elements parameter uint8; ECUAPPM_CONTEXTFLAG parameter uint8; ECUAPPM_MIN_GROUP_ACTIVE_TIME parameter uint16; EcuAppMActivationTimer local uint16; ECUAPPM_GROUP_ACTIVATION_TYPE parameter uint8
